simulink model "Compliant_inboard_steering_model"  (R2020b)
settings: Solver=VariableStepAuto  StartTime=0.0  StopTime=10.0  RelTol=1e-3
values from neighbouring files (symbols this model uses):
  steer =     [Compliat_inboard_steering_workspace.mat]
libraries: pid_lib x1
settings Model: Creator=Jon  LastModifiedBy=Jon

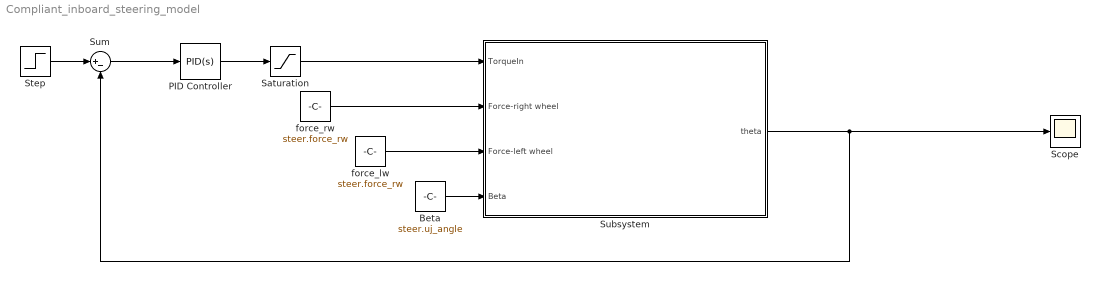
== system Compliant_inboard_steering_model ==
  Beta : Constant  Value=steer.uj_angle
  PID Controller : pid_lib/PID Controller  Controller=PID  Form=Parallel  TimeDomain=Continuous-time  UseExternalTs=off  SampleTime=-1  IntegratorMethod=Forward Euler  FilterMethod=Forward Euler  ControllerParametersSource=internal  P=1  I=1  D=0  UseFilter=on  N=100  TunerSelectOption=Transfer Function Based (PID Tuner App)  InitialConditionSource=internal  InitialConditionForIntegrator=0  InitialConditionForFilter=0  DifferentiatorICPrevScaledInput=0  ExternalReset=none  TrackingMode=off  Kt=1  LimitOutput=off  SatLimitsSource=internal  UpperSaturationLimit=inf  LowerSaturationLimit=-inf  LinearizeAsGain=on  AntiWindupMode=none  Kb=1  POutMin=[]  POutMax=[]  IOutMin=[]  IOutMax=[]  DOutMin=[]  DOutMax=[]  NOutMin=[]  NOutMax=[]  SumOutMin=[]  SumOutMax=[]  SaturationOutMin=[]  SaturationOutMax=[]  PParamMin=[]  PParamMax=[]  IParamMin=[]  IParamMax=[]  DParamMin=[]  DParamMax=[]  NParamMin=[]  NParamMax=[]  KbParamMin=[]  KbParamMax=[]  KtParamMin=[]  KtParamMax=[]  KbOutMin=[]  KbOutMax=[]  KtOutMin=[]  KtOutMax=[]  IntegratorOutMin=[]  IntegratorOutMax=[]  FilterOutMin=[]  FilterOutMax=[]  SumI1OutMin=[]  SumI1OutMax=[]  SumI2OutMin=[]  SumI2OutMax=[]  SumI3OutMin=[]  SumI3OutMax=[]  SumI4OutMin=[]  SumI4OutMax=[]  SumDOutMin=[]  SumDOutMax=[]  DifferentiatorOutMin=[]  DifferentiatorOutMax=[]  FilterDiffOutCoefMin=[]  FilterDiffOutCoefMax=[]  ReciprocalOutMin=[]  ReciprocalOutMax=[]  SumDenOutMin=[]  SumDenOutMax=[]  SumNumOutMin=[]  SumNumOutMax=[]  DivideOutMin=[]  DivideOutMax=[]  UdiffTsProdOutMin=[]  UdiffTsProdOutMax=[]  NTsProdOutMin=[]  NTsProdOutMax=[]  UintegralTsProdOutMin=[]  UintegralTsProdOutMax=[]  UngainTsProdOutMin=[]  UngainTsProdOutMax=[]  IntegratorContinuousStateAttributes=''  IntegratorStateMustResolveToSignalObject=off  IntegratorRTWStateStorageClass=Auto  FilterContinuousStateAttributes=''  FilterStateMustResolveToSignalObject=off  FilterRTWStateStorageClass=Auto  ParallelPVariant=InternalParameters  IdealPVariant=Disabled  IVariant=InternalParameters  DVariant=InternalParameters  IntegratorVariant=Continuous  SatVariant=Disabled  AWVariant=Passthrough  PCopyVariant=Disabled  TRVariant=Disabled  FdbkBlocksVariant=Forward  IdealPFdbkVariant=Disabled  SatFdbkVariant=Disabled  DerivativeFilterVariant=ContFilter  NVariant=InternalParameters  NCopyVariant=Disabled  FilterICVariant=InternalICsFilter  IntegratorICVariant=InternalICs  ExternalResetVariant=Disabled  TRSumVariant=Passthrough  SumFdbkVariant=Disabled  SumVariant=Sum_PID  TsampFilterVariant=InternalTs  TsampNgainVariant=Passthrough  TsampIntegralVariant=Passthrough  ExternalSaturationOutDataTypeStr=Inherit: Same as second input
  Saturation : Saturate
  Scope : Scope
  Step : Step  SampleTime=0
  Subsystem : Subsystem
  Sum : Sum  Inputs=|+-
  force_lw : Constant  Value=steer.force_rw
  force_rw : Constant  Value=steer.force_rw
  wires:
  Step/1 -> Sum/1
  PID Controller/1 -> Saturation/1
  Saturation/1 -> Subsystem/1(TorqueIn)
  force_rw/1 -> Subsystem/2(Force-right wheel)
  force_lw/1 -> Subsystem/3(Force-left wheel)
  Beta/1 -> Subsystem/4(Beta)
  Subsystem/1(theta) -> Sum/2, Scope/1
  Sum/1 -> PID Controller/1

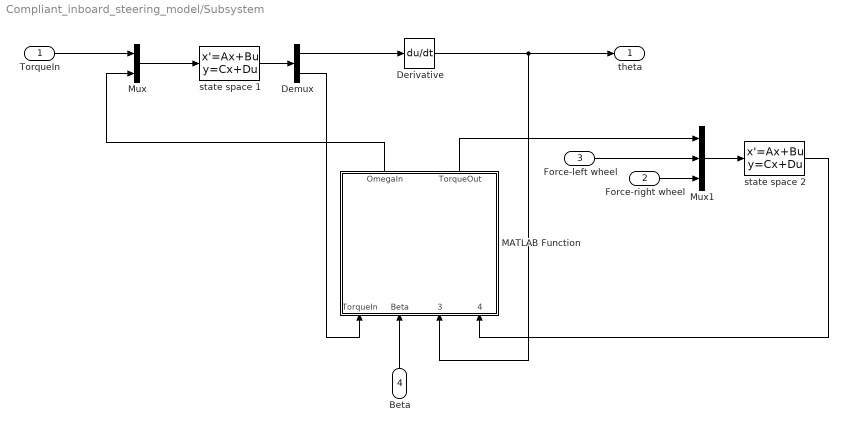
== system Compliant_inboard_steering_model/Subsystem ==
  TorqueIn : Inport
  Force-right wheel : Inport  Port=2
  Force-left wheel : Inport  Port=3
  Beta : Inport  Port=4
  Demux : Demux  Outputs=2
  Derivative : Derivative
  MATLAB Function : MATLAB Function  TreatAsAtomicUnit=on
  Mux : Mux  Inputs=2
  Mux1 : Mux  Inputs=3
  state space 1 : StateSpace  A=[0,-steer.compliance.k_sw; 1/steer.inertia.j_sw,0]  B=[1,0 ; 0,-1]  C="[1/steer.inertia.j_sw , 0     ;  0 , steer.compliance.q_sw]"  D=[0,0;0,0]  InitialCondition=0  ContinuousStateAttributes=1st state space
  state space 2 : StateSpace  A="[0 , -steer.compliance.k_sc , 0;  1/steer.inertia.j_sw, 0 , -2*pi/(steer.rack.c*steer.inertia.m_r); 0, 2*pi/(steer.rack.c*steer.compliance.k_sc),-steer.resistance.b/steer.inertia.m_r]"  B=[1,0,0;0,0,0;0,-1,-1]  C=[1/steer.inertia.j_sc,0,0]  D=[0,0,0]  InitialCondition=0
  theta : Outport
  wires:
  TorqueIn/1 -> Mux/1
  MATLAB Function/1(OmegaIn) -> Mux/2
  Mux/1 -> state space 1/1
  state space 1/1 -> Demux/1
  Mux1/1 -> state space 2/1
  Force-right wheel/1 -> Mux1/3
  Force-left wheel/1 -> Mux1/2
  Demux/2 -> MATLAB Function/1(TorqueIn)
  Demux/1 -> Derivative/1
  Derivative/1 -> MATLAB Function/3(ThetaOut), theta/1
  Beta/1 -> MATLAB Function/2(Beta)
  state space 2/1 -> MATLAB Function/4(OmegaOut)
  MATLAB Function/2(TorqueOut) -> Mux1/1

== matlab function Compliant_inboard_steering_model/Subsystem/MATLAB Function ==
  data: TorqueIn input; Beta input; ThetaOut input; OmegaIn output; TorqueOut output; OmegaOut input
function [OmegaIn, TorqueOut] = CardenTransformation(TorqueIn,Beta,ThetaOut,OmegaOut)

OmegaIn = OmegaOut .* cosd(Beta) ./ ( 1 - (sind(Beta).*cos(ThetaOut)).^2 );

TorqueOut = TorqueIn .* cosd(Beta) ./ ( 1 - (sind(Beta).*cos(ThetaOut)).^2 );
